simulink library "FDI"  (R2017b)
settings: Solver=VariableStepAuto  StartTime=0.0  StopTime=10.0  RelTol=1e-3
undefined symbols (not defined in the file or in its folder): A, B, Blat1, BWBlat, rho, T, x0
libraries: dspinverses x1, dspmtrx3 x1
settings Model: Creator=Liam Uni  LastModifiedBy=Liam Uni

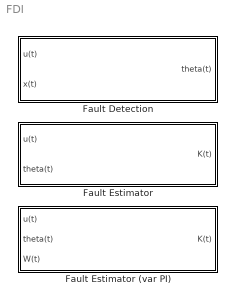
== system FDI ==
  Fault Detection : Subsystem  mask{A=A, B=B, x0=x0, rho=rho, delta=0, eps=0}
      mask prompts: A "System Matrix (A)"; B "Effectiveness Matrix (B)"; x0 "Initial State (x0)"
      mask init:
      | Gn=eye(size(A,1))
      mask DialogControl DescGroupVar Prompt: Fault Detection Unit
      mask DialogControl DescTextVar Prompt: During ideal sliding theta(t)~=-BKu(t). A sigmoidal function can be used to create a continuous pseudo-sliding non-linear component using delta: sig(s)=P2s/(||P2s||+delta).  A boundary layer around the sliding surface can be used using eps: if ||P2s||>eps un(t)=un(t) if ||P2s||<=eps un(t)=0
      mask DialogControl Container4 Prompt: Model Parameters
      mask DialogControl Container5 Prompt: Controller Parameters
      mask DialogControl Container6 Prompt: Gain Tuning
      mask DialogControl Container7 Prompt: Chattering Avoidance
      mask Display:
      | disp('Fault Detection')
      | port_label('input', 1, 'x(t)');
      | port_label('input', 2, 'u(t)');
      | port_label('output', 1, 'theta(t)');
  Fault Estimator : Subsystem  mask{B=B, T=T, eps=eps}
      mask prompts: B "Effectiveness Matrix (B)"; T "Zero-order hold constant"
      mask DialogControl DescGroupVar Prompt: Fault Estimator
      mask DialogControl DescTextVar Prompt: Calculates an approximate value of K(t) from theta(t)=-BK(t)u(t)
      mask Display:
      | disp('Fault Estimator')
      | port_label('input', 1, 'u(t)');
      | port_label('input', 2, 'theta(t)');
      | port_label('output', 1, 'K(t)');
  Fault Estimator (var PI) : Subsystem  mask{B=B, T=T, eps=eps}
      mask prompts: B "Effectiveness Matrix (B)"; T "Zero-order hold constant"
      mask DialogControl DescGroupVar Prompt: Fault Estimator
      mask DialogControl DescTextVar Prompt: Calculates an approximate value of K(t) from theta(t)=-BK(t)u(t). The signal W(t) is used to vary the pseudo-inverse of B.
      mask Display:
      | disp('Fault Estimator (var PI)')
      | port_label('input', 1, 'u(t)');
      | port_label('input', 2, 'theta(t)');
      | port_label('input', 3, 'W(t)');
      | port_label('output', 1, 'K(t)');

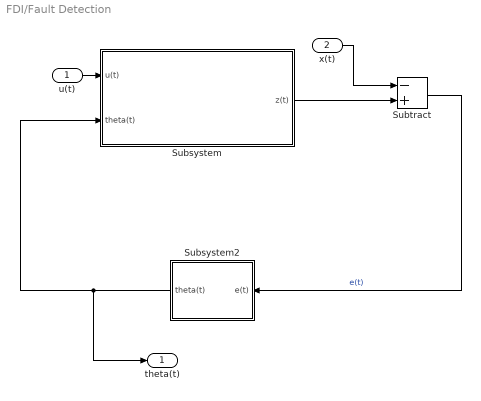
== system FDI/Fault Detection ==
  u(t) : Inport
  x(t) : Inport  Port=2
  Subsystem : Subsystem
  Subsystem2 : Subsystem
  Subtract : Sum  Inputs=-+
  theta(t) : Outport
  wires:
  x(t)/1 -> Subtract/1
  u(t)/1 -> Subsystem/1(u(t))
  Subsystem2/1(theta(t)) -> theta(t)/1, Subsystem/2(theta(t))
  Subtract/1 -> Subsystem2/1(e(t))  "e(t)"
  Subsystem/1(z(t)) -> Subtract/2

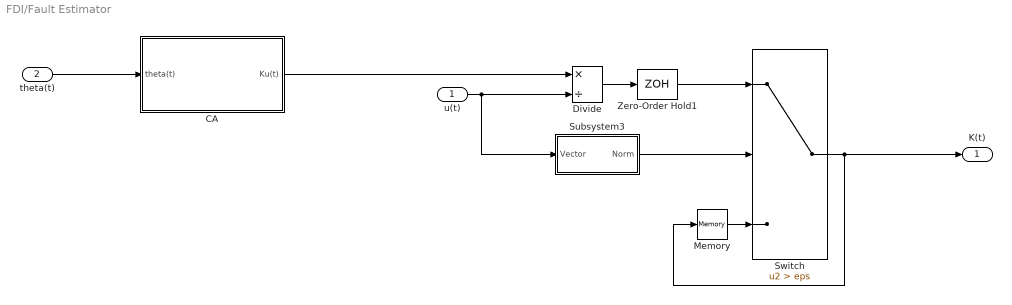
== system FDI/Fault Estimator ==
  u(t) : Inport
  theta(t) : Inport  Port=2
  CA : Subsystem
  Divide : Product  Inputs=*/
  Memory : Memory
  Subsystem3 : Subsystem
  Switch : Switch  Criteria=u2 > Threshold  Threshold=eps
  Zero-Order Hold1 : ZeroOrderHold  SampleTime=T
  K(t) : Outport
  wires:
  u(t)/1 -> Subsystem3/1(Vector), Divide/2
  Divide/1 -> Zero-Order Hold1/1
  CA/1("Ku(t) ") -> Divide/1
  Zero-Order Hold1/1 -> Switch/1
  theta(t)/1 -> CA/1(theta(t))
  Subsystem3/1(Norm) -> Switch/2
  Switch/1 -> Memory/1, K(t)/1
  Memory/1 -> Switch/3

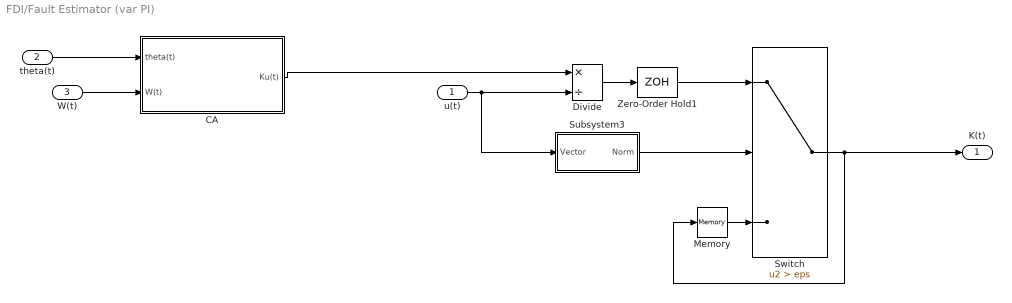
== system FDI/Fault Estimator (var PI) ==
  u(t) : Inport
  theta(t) : Inport  Port=2
  W(t) : Inport  Port=3
  CA : Subsystem
  Divide : Product  Inputs=*/
  Memory : Memory
  Subsystem3 : Subsystem
  Switch : Switch  Criteria=u2 > Threshold  Threshold=eps
  Zero-Order Hold1 : ZeroOrderHold  SampleTime=T
  K(t) : Outport
  wires:
  u(t)/1 -> Subsystem3/1(Vector), Divide/2
  Divide/1 -> Zero-Order Hold1/1
  CA/1("Ku(t) ") -> Divide/1
  Zero-Order Hold1/1 -> Switch/1
  theta(t)/1 -> CA/1(theta(t))
  Subsystem3/1(Norm) -> Switch/2
  Switch/1 -> Memory/1, K(t)/1
  Memory/1 -> Switch/3
  W(t)/1 -> CA/2(W(t))

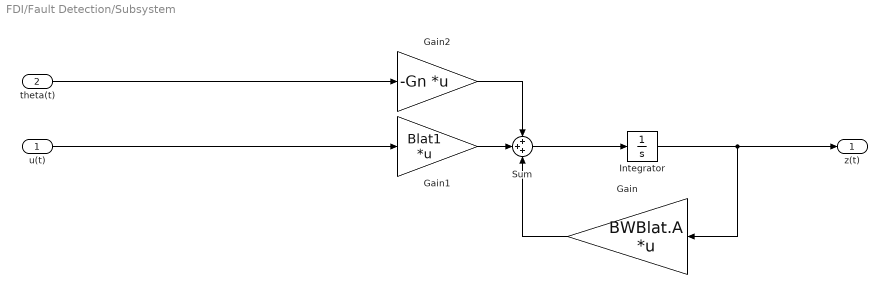
== system FDI/Fault Detection/Subsystem ==
  u(t) : Inport
  theta(t) : Inport  Port=2
  Gain : Gain  Gain=BWBlat.A  Multiplication=Matrix(K*u) (u vector)
  Gain1 : Gain  Gain=Blat1  Multiplication=Matrix(K*u) (u vector)
  Gain2 : Gain  Gain=-Gn  Multiplication=Matrix(K*u) (u vector)
  Integrator : Integrator  InitialCondition=x0
  Sum : Sum  Inputs=+++
  z(t) : Outport
  wires:
  Gain1/1 -> Sum/2
  theta(t)/1 -> Gain2/1
  Gain2/1 -> Sum/1
  Sum/1 -> Integrator/1
  u(t)/1 -> Gain1/1
  Integrator/1 -> z(t)/1, Gain/1
  Gain/1 -> Sum/3

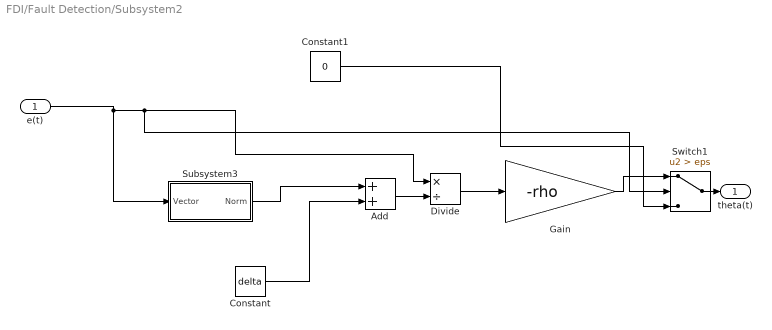
== system FDI/Fault Detection/Subsystem2 ==
  e(t) : Inport
  Add : Sum
  Constant : Constant  Value=delta
  Constant1 : Constant  Value=0
  Divide : Product  Inputs=*/
  Gain : Gain  Gain=-rho
  Subsystem3 : Subsystem
  Switch1 : Switch  Criteria=u2 > Threshold  Threshold=eps  ZeroCross=off
  theta(t) : Outport
  wires:
  Subsystem3/1(Norm) -> Add/1
  Add/1 -> Divide/2
  Constant/1 -> Add/2
  Divide/1 -> Gain/1
  Gain/1 -> Switch1/1
  e(t)/1 -> Subsystem3/1(Vector), Switch1/2, Divide/1
  Constant1/1 -> Switch1/3
  Switch1/1 -> theta(t)/1

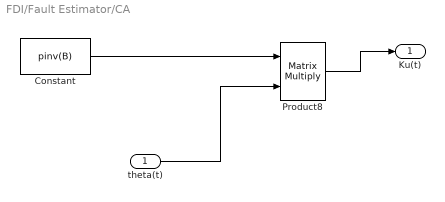
== system FDI/Fault Estimator/CA ==
  theta(t) : Inport
  Constant : Constant  Value=pinv(B)
  Product8 : Product  Multiplication=Matrix(*)
  "Ku(t) " : Outport
  wires:
  Product8/1 -> "Ku(t) "/1
  theta(t)/1 -> Product8/2
  Constant/1 -> Product8/1

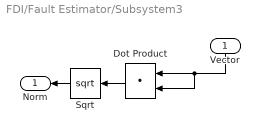
== system FDI/Fault Estimator/Subsystem3 ==
  Vector : Inport
  Dot Product : DotProduct  InputSameDT=on  OutDataTypeStr=Inherit: Inherit via internal rule
  Sqrt : Sqrt  SaturateOnIntegerOverflow=on
  Norm : Outport
  wires:
  Vector/1 -> Dot Product/1, Dot Product/2
  Sqrt/1 -> Norm/1
  Dot Product/1 -> Sqrt/1

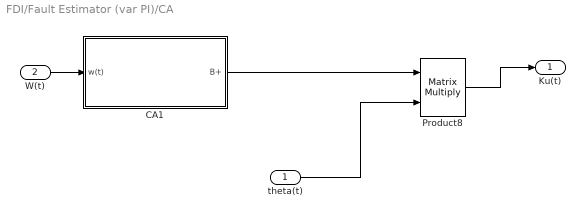
== system FDI/Fault Estimator (var PI)/CA ==
  theta(t) : Inport
  W(t) : Inport  Port=2
  CA1 : Subsystem
  Product8 : Product  Multiplication=Matrix(*)
  "Ku(t) " : Outport
  wires:
  Product8/1 -> "Ku(t) "/1
  theta(t)/1 -> Product8/2
  CA1/1("B+ ") -> Product8/1
  W(t)/1 -> CA1/1(w(t))

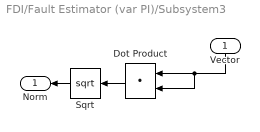
== system FDI/Fault Estimator (var PI)/Subsystem3 ==
  Vector : Inport
  Dot Product : DotProduct  InputSameDT=on  OutDataTypeStr=Inherit: Inherit via internal rule
  Sqrt : Sqrt  SaturateOnIntegerOverflow=on
  Norm : Outport
  wires:
  Vector/1 -> Dot Product/1, Dot Product/2
  Sqrt/1 -> Norm/1
  Dot Product/1 -> Sqrt/1

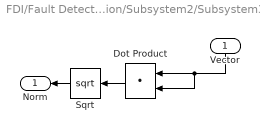
== system FDI/Fault Detection/Subsystem2/Subsystem3 ==
  Vector : Inport
  Dot Product : DotProduct  InputSameDT=on  OutDataTypeStr=Inherit: Inherit via internal rule
  Sqrt : Sqrt  SaturateOnIntegerOverflow=on
  Norm : Outport
  wires:
  Vector/1 -> Dot Product/1, Dot Product/2
  Sqrt/1 -> Norm/1
  Dot Product/1 -> Sqrt/1

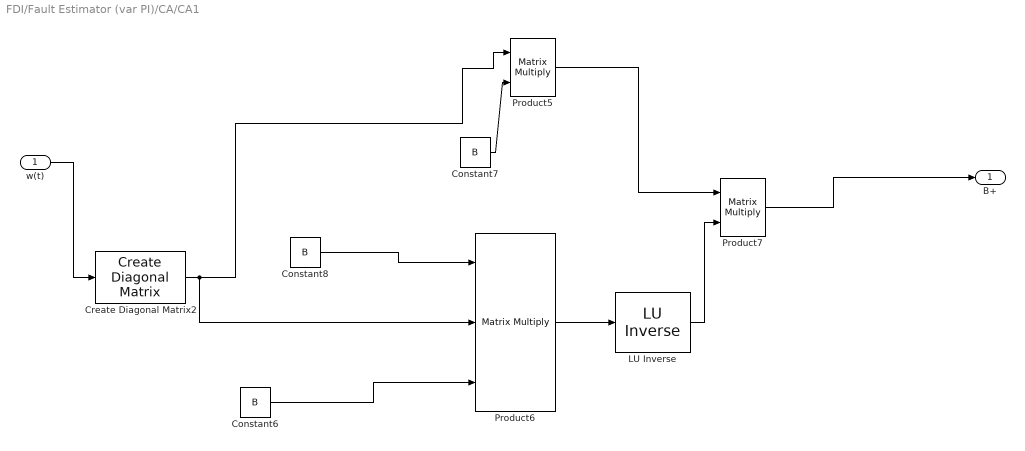
== system FDI/Fault Estimator (var PI)/CA/CA1 ==
  w(t) : Inport
  " LU Inverse" : dspinverses/ LU Inverse
      settings: SourceProductName=DSP System Toolbox
  Constant6 : Constant  Value=B
  Constant7 : Constant  Value=B
  Constant8 : Constant  Value=B
  Create Diagonal Matrix2 : dspmtrx3/Create Diagonal Matrix
      settings: SourceProductName=DSP System Toolbox  SourceProductBaseCode=DS
  Product5 : Product  Multiplication=Matrix(*)
  Product6 : Product  Inputs=3  Multiplication=Matrix(*)
  Product7 : Product  Multiplication=Matrix(*)
  "B+ " : Outport
  wires:
  Create Diagonal Matrix2/1 -> Product6/2, Product5/1
  Product5/1 -> Product7/1
  Constant8/1 -> Product6/1
  Constant6/1 -> Product6/3
  Constant7/1 -> Product5/2
  w(t)/1 -> Create Diagonal Matrix2/1
  Product7/1 -> "B+ "/1
  Product6/1 -> " LU Inverse"/1
  " LU Inverse"/1 -> Product7/2
